simulink model "k1visbsp"  (Simulink 8.6)
settings: Solver=ode45  StartTime=0.0  StopTime=10.0  RelTol=1e-3
libraries: cdsEpicsOut x53, cdsTP x48, cdsFilt x30, cdsFiltCtrl x24, cdsEpicsStringIn x24, cdsRms x24, cdsIPCx x15, STATE_BIO_MASTER x3, cdsCDI64 x3, cdsCDO64 x3, VIS_LIB x2, cdsMuxMatrix x2
(part 1 of 4)
settings Model: Creator=controls  LastModifiedBy=controls
settings DataIOCC: SignalLoggingSaveFormat=Dataset
settings OptimizationCC: ExpressionDepthLimit=128
settings DebuggingCC: UnderspecifiedInitializationDetection=Simplified  MergeDetectMultiDrivingBlocksExec=error  SolverPrmCheckMsg=none  FcnCallInpInsideContextMsg=EnableAllAsError  StateNameClashWarn=none
settings GRTTargetCC: CombineOutputUpdateFcns=on  GRTInterface=off

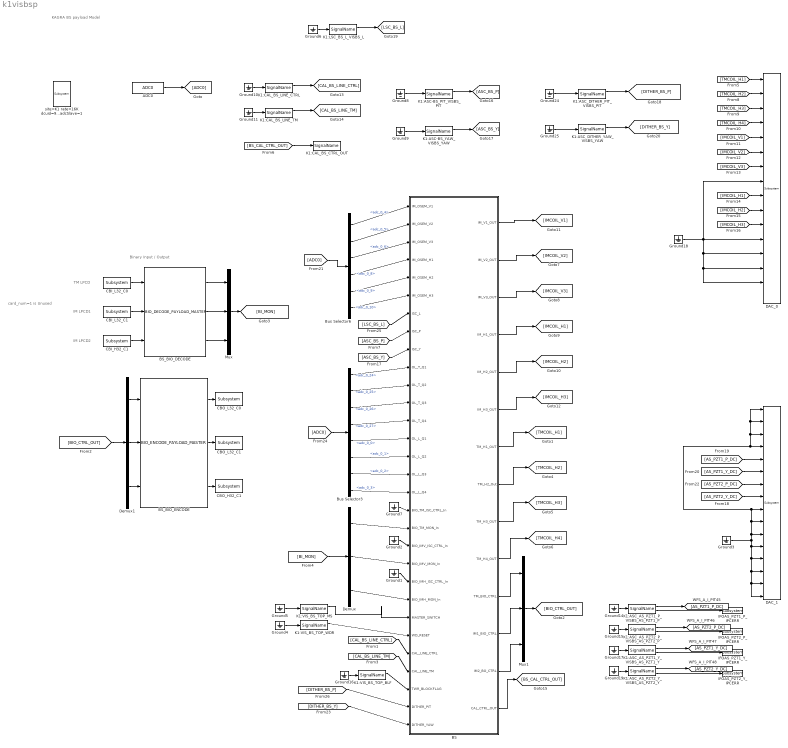
== system k1visbsp ==
  note: KAGRA BS payload Model
  note: TM LPCD
  note: Binary Input / Output
  note: card_num=1 is Unused
  note: IM LPCD1
  note: IM LPCD2
  ADC0 : cdsAdcx0/ADC0  Tag=cdsAdc  Description=|
      | type-GSC_16AI64SSA
      | card_num=0
      settings: AttributesFormatString=%<Description>\n%<Tag>
  BS : Subsystem  AncestorBlock=TYPEB_MASTER/TYPEB_PAYLOAD_shutdown
  BS_BIO_DECODE : TYPEB_MASTER/BIO_DECODE_PAYLOAD_MASTER
  BS_BIO_ENCODE : TYPEB_MASTER/BIO_ENCODE_PAYLOAD_MASTER
  Bus Selector3 : BusSelector  Description=ADC Selector  OutputSignals=adc_0_24,adc_0_25,adc_0_26,adc_0_27,adc_0_0,adc_0_1,adc_0_2,adc_0_3
      settings: AttributesFormatString=%<Description>
  Bus Selector6 : BusSelector  Description=ADC Selector  OutputSignals=adc_0_4,adc_0_5,adc_0_6,adc_0_8,adc_0_9,adc_0_10
      settings: AttributesFormatString=%<Description>
  CBI_H32_C1 : cdsCDI64/Subsystem  Tag=cdsCDI64  Description=card_num=3
      settings: AttributesFormatString=%<Tag>\n%<Description>
  CBI_L32_C0 : cdsCDI64/Subsystem  Tag=cdsCDI64  Description=card_num=0
      settings: AttributesFormatString=%<Tag>\n%<Description>
  CBI_L32_C1 : cdsCDI64/Subsystem  Tag=cdsCDI64  Description=card_num=2
      settings: AttributesFormatString=%<Tag>\n%<Description>
  CBO_H32_C1 : cdsCDO64/Subsystem  Tag=cdsCDO64  Description=card_num=3
      settings: AttributesFormatString=%<Tag>\n%<Description>
  CBO_L32_C0 : cdsCDO64/Subsystem  Tag=cdsCDO64  Description=card_num=0
      settings: AttributesFormatString=%<Tag>\n%<Description>
  CBO_L32_C1 : cdsCDO64/Subsystem  Tag=cdsCDO64  Description=card_num=2
      settings: AttributesFormatString=%<Tag>\n%<Description>
  DAC_0 : dac/Subsystem  Description=|
      | type=GSC_16AO16,
      | card_num=0
      settings: AttributesFormatString=%<Description>
  DAC_1 : dac/Subsystem  Description=|
      | type=GSC_16AO16,
      | card_num=1
      settings: AttributesFormatString=%<Description>
  Demux : Demux  Outputs=3
  Demux1 : Demux  Outputs=3
  Ground{1..11,14..19,24..25} (19 alike) : Ground
  IFOAS_PZT1_P_IPCERR : cdsEpicsOut/Subsystem  Tag=cdsEpicsOutput  Description=|
      | Purpose:                                          
      | Output a FE signal to an EPICS channel.           
      |                                                   
      | Operation:                                        
      | Takes input value and passes it to EPICS record.  
      |                                                   
      | Usage:                                            
      | Name the part with the desired EPICS rrecord name.
      settings: AttributesFormatString=%<Tag>
  IFOAS_PZT1_Y_IPCERR : cdsEpicsOut/Subsystem  Tag=cdsEpicsOutput  Description=|
      | Purpose:                                          
      | Output a FE signal to an EPICS channel.           
      |                                                   
      | Operation:                                        
      | Takes input value and passes it to EPICS record.  
      |                                                   
      | Usage:                                            
      | Name the part with the desired EPICS rrecord name.
      settings: AttributesFormatString=%<Tag>
  IFOAS_PZT2_P_IPCERR : cdsEpicsOut/Subsystem  Tag=cdsEpicsOutput  Description=|
      | Purpose:                                          
      | Output a FE signal to an EPICS channel.           
      |                                                   
      | Operation:                                        
      | Takes input value and passes it to EPICS record.  
      |                                                   
      | Usage:                                            
      | Name the part with the desired EPICS rrecord name.
      settings: AttributesFormatString=%<Tag>
  IFOAS_PZT2_Y_IPCERR : cdsEpicsOut/Subsystem  Tag=cdsEpicsOutput  Description=|
      | Purpose:                                          
      | Output a FE signal to an EPICS channel.           
      |                                                   
      | Operation:                                        
      | Takes input value and passes it to EPICS record.  
      |                                                   
      | Usage:                                            
      | Name the part with the desired EPICS rrecord name.
      settings: AttributesFormatString=%<Tag>
  K1:ASC-BS_PIT_VISBS_PIT : cdsIPCx/SignalName  Tag=cdsIPCx_PCIE  Description=Inter-Process Communication via PCI Express network.
      settings: AttributesFormatString=%<Tag>
  K1:ASC-BS_YAW_VISBS_YAW : cdsIPCx/SignalName  Tag=cdsIPCx_PCIE  Description=Inter-Process Communication via PCI Express network.
      settings: AttributesFormatString=%<Tag>
  K1:ASC_AS_PZT1_P_VISBS_AS_PZT1_P : cdsIPCx/SignalName  Tag=cdsIPCx_PCIE  Description=Inter-Process Communication via PCI Express network.
      settings: AttributesFormatString=%<Tag>
  K1:ASC_AS_PZT1_Y_VISBS_AS_PZT1_Y : cdsIPCx/SignalName  Tag=cdsIPCx_PCIE  Description=Inter-Process Communication via PCI Express network.
      settings: AttributesFormatString=%<Tag>
  K1:ASC_AS_PZT2_P_VISBS_AS_PZT2_P : cdsIPCx/SignalName  Tag=cdsIPCx_PCIE  Description=Inter-Process Communication via PCI Express network.
      settings: AttributesFormatString=%<Tag>
  K1:ASC_AS_PZT2_Y_VISBS_AS_PZT2_Y : cdsIPCx/SignalName  Tag=cdsIPCx_PCIE  Description=Inter-Process Communication via PCI Express network.
      settings: AttributesFormatString=%<Tag>
  K1:ASC_DITHER_PIT_VISBS_PIT : cdsIPCx/SignalName  Tag=cdsIPCx_PCIE  Description=Inter-Process Communication via PCI Express network.
      settings: AttributesFormatString=%<Tag>
  K1:ASC_DITHER_YAW_VISBS_YAW : cdsIPCx/SignalName  Tag=cdsIPCx_PCIE  Description=Inter-Process Communication via PCI Express network.
      settings: AttributesFormatString=%<Tag>
  K1:CAL_BS_CTRL_OUT : cdsIPCx/SignalName  Tag=cdsIPCx_PCIE  Description=Inter-Process Communication via PCI Express network.
      settings: AttributesFormatString=%<Tag>
  K1:CAL_BS_LINE_CTRL : cdsIPCx/SignalName  Tag=cdsIPCx_PCIE  Description=Inter-Process Communication via PCI Express network.
      settings: AttributesFormatString=%<Tag>
  K1:CAL_BS_LINE_TM : cdsIPCx/SignalName  Tag=cdsIPCx_PCIE  Description=Inter-Process Communication via PCI Express network.
      settings: AttributesFormatString=%<Tag>
  K1:LSC_BS_L_VISBS_L : cdsIPCx/SignalName  Tag=cdsIPCx_PCIE  Description=Inter-Process Communication via PCI Express network.
      settings: AttributesFormatString=%<Tag>
  K1:VIS_BS_TOP_BLF : cdsIPCx/SignalName  Tag=cdsIPCx_SHMEM  Description=Inter-Process Communication via Shared memory.
      settings: AttributesFormatString=%<Tag>
  K1:VIS_BS_TOP_MS : cdsIPCx/SignalName  Tag=cdsIPCx_SHMEM  Description=Inter-Process Communication via Shared memory.
      settings: AttributesFormatString=%<Tag>
  K1:VIS_BS_TOP_WDR : cdsIPCx/SignalName  Tag=cdsIPCx_SHMEM  Description=Inter-Process Communication via Shared memory.
      settings: AttributesFormatString=%<Tag>
  Mux : Mux  Inputs=3
  Mux1 : Mux  Inputs=3
  site=K1 rate=16K dcuid=92 host=k1bs specific_cpu=5 adcSlave=1 : cdsParameters/Subsystem  Tag=cdsParameters  Description=|
      | Purpose:                                                                                                                                                                                                                                
      | Provide system parameters to the FE code generator to properly configure the generated EPICS names, rep rate of the FE controller, and the Data Acquisition node ID for proper storage of data from this FE controller.                 
      |                                                                                                                                                                                                                                         
      | Useage:                                                                                                                                                                                                                                 
      | The part NAME field is used to identify the FE parameters. It must be of the form:                                                                                                                                                      
      | site=                                                                                                                                                                                                                                   
      | rate=                                                                                                                                                                                                                                   
      | dcuid=                                                                                                                                                                                                                                  
      |                                                                                                                                                                                                                                         
      | Where:                                                                                                                                                                                                                                  
      | site= argument may be H1, H2, L1, M1, G1, either as a single argument or multiple, for example site=H1,H2. These are the only names allowed. These will become the first two characters of all EPICS and signal names (for example G1:).
      |                                                                                                                                                                                                                                         
      | rate= may be 2K, 16K, 32K, or 64K                                                                                                                                                                                                       
      |                                                                                                                                                                                                                                         
      | dcuid= is site specific ie it must be unique at each site.
      settings: AttributesFormatString=%<Tag>
  wires:
  ADC0/1 -> [ADC0]
  [ADC0] -> Bus Selector6/1
  BS/10(TM_H4_OUT) -> [TMCOIL_H4]
  BS/9(TM_H3_OUT) -> [TMCOIL_H3]
  BS/8(TM_H2_Out) -> [TMCOIL_H2]
  BS/7(TM_H1_OUT) -> [TMCOIL_H1]
  BS/1(IM_V1_OUT) -> [IMCOIL_V1]
  BS/2(IM_V2_OUT) -> [IMCOIL_V2]
  BS/3(IM_V3_OUT) -> [IMCOIL_V3]
  BS/4(IM_H1_OUT) -> [IMCOIL_H1]
  BS/5(IM_H2_OUT) -> [IMCOIL_H2]
  BS/6(IM_H3_OUT) -> [IMCOIL_H3]
  Ground18/1 -> DAC_0/12, DAC_0/13, DAC_0/14, DAC_0/15, DAC_0/8
  Bus Selector6/1 -> BS/1(IM_OSEM_V1)  "<adc_0_4>"
  Bus Selector6/2 -> BS/2(IM_OSEM_V2)  "<adc_0_5>"
  Bus Selector6/3 -> BS/3(IM_OSEM_V3)  "<adc_0_6>"
  [TMCOIL_H2] -> DAC_0/2
  [TMCOIL_H3] -> DAC_0/3
  [TMCOIL_H1] -> DAC_0/1
  [TMCOIL_H4] -> DAC_0/4
  [IMCOIL_V1] -> DAC_0/5
  [IMCOIL_V2] -> DAC_0/6
  [IMCOIL_V3] -> DAC_0/7
  Bus Selector6/4 -> BS/4(IM_OSEM_H1)  "<adc_0_8>"
  Bus Selector6/5 -> BS/5(IM_OSEM_H2)  "<adc_0_9>"
  Bus Selector6/6 -> BS/6(IM_OSEM_H3)  "<adc_0_10>"
  [IMCOIL_H3] -> DAC_0/11
  [IMCOIL_H2] -> DAC_0/10
  [IMCOIL_H1] -> DAC_0/9
  [LSC_BS_L] -> BS/7(ISC_L)
  [ADC0] -> Bus Selector3/1
  Bus Selector3/1 -> BS/10(OL_T_Q1)  "<adc_0_24>"
  Bus Selector3/2 -> BS/11(OL_T_Q2)  "<adc_0_25>"
  Bus Selector3/3 -> BS/12(OL_T_Q3)  "<adc_0_26>"
  Bus Selector3/4 -> BS/13(OL_T_Q4)  "<adc_0_27>"
  BS_BIO_ENCODE/1 -> CBO_L32_C0/1
  BS_BIO_ENCODE/3 -> CBO_H32_C1/1
  BS_BIO_ENCODE/2 -> CBO_L32_C1/1
  CBI_L32_C0/1 -> BS_BIO_DECODE/1
  CBI_L32_C1/1 -> BS_BIO_DECODE/2
  CBI_H32_C1/1 -> BS_BIO_DECODE/3
  BS_BIO_DECODE/2 -> Mux/2
  BS_BIO_DECODE/3 -> Mux/3
  BS_BIO_DECODE/1 -> Mux/1
  Mux/1 -> [BI_MON]
  Demux1/2 -> BS_BIO_ENCODE/2
  Demux1/3 -> BS_BIO_ENCODE/3
  Demux1/1 -> BS_BIO_ENCODE/1
  [BIO_CTRL_OUT] -> Demux1/1
  Mux1/1 -> [BIO_CTRL_OUT]
  [BI_MON] -> Demux/1
  Demux/1 -> BS/19(BIO_TM_MON_In)
  Demux/2 -> BS/21(BIO_IMV_MON_In)
  Demux/3 -> BS/23(BIO_IMH_MON_In)
  Ground7/1 -> BS/18(BIO_TM_ISC_CTRL_In)
  Ground1/1 -> BS/22(BIO_IMH_ISC_CTRL_In)
  Ground2/1 -> BS/20(BIO_IMV_ISC_CTRL_In)
  Ground4/1 -> K1:VIS_BS_TOP_WDR/1
  Ground5/1 -> K1:VIS_BS_TOP_MS/1
  K1:VIS_BS_TOP_WDR/1 -> BS/25(WD_RESET)
  K1:VIS_BS_TOP_MS/1 -> BS/24(MASTER_SWITCH)
  Ground10/1 -> K1:CAL_BS_LINE_CTRL/1
  K1:CAL_BS_LINE_CTRL/1 -> [CAL_BS_LINE_CTRL]
  Ground11/1 -> K1:CAL_BS_LINE_TM/1
  K1:CAL_BS_LINE_TM/1 -> [CAL_BS_LINE_TM]
  [CAL_BS_LINE_CTRL] -> BS/26(CAL_LINE_CTRL)
  [CAL_BS_LINE_TM] -> BS/27(CAL_LINE_TM)
  BS/14(CAL_CTRL_OUT) -> [BS_CAL_CTRL_OUT]
  [BS_CAL_CTRL_OUT] -> K1:CAL_BS_CTRL_OUT/1
  Ground3/1 -> DAC_1/13, DAC_1/14, DAC_1/15, DAC_1/16, DAC_1/12, DAC_1/1, DAC_1/2, DAC_1/3, DAC_1/4, DAC_1/9, DAC_1/10, DAC_1/11
  Bus Selector3/5 -> BS/14(OL_L_Q1)  "<adc_0_0>"
  Bus Selector3/6 -> BS/15(OL_L_Q2)  "<adc_0_1>"
  Bus Selector3/7 -> BS/16(OL_L_Q3)  "<adc_0_2>"
  Bus Selector3/8 -> BS/17(OL_L_Q4)  "<adc_0_3>"
  [ASC_BS_P] -> BS/8(ISC_P)
  [ASC_BS_Y] -> BS/9(ISC_Y)
  Ground16/1 -> K1:VIS_BS_TOP_BLF/1
  K1:VIS_BS_TOP_BLF/1 -> BS/28(TWR_BLOCKFLAG)
  BS/11(TM_BIO_CTRL) -> Mux1/1
  BS/12(IM1_BIO_CTRL) -> Mux1/2
  BS/13(IM2_BO_CTRL) -> Mux1/3
  [DITHER_BS_Y] -> BS/30(DITHER_YAW)
  K1:ASC_AS_PZT1_P_VISBS_AS_PZT1_P/2 -> IFOAS_PZT1_P_IPCERR/1
  K1:ASC_AS_PZT2_P_VISBS_AS_PZT2_P/2 -> IFOAS_PZT2_P_IPCERR/1
  K1:ASC_AS_PZT1_Y_VISBS_AS_PZT1_Y/2 -> IFOAS_PZT1_Y_IPCERR/1
  K1:ASC_AS_PZT2_Y_VISBS_AS_PZT2_Y/2 -> IFOAS_PZT2_Y_IPCERR/1
  K1:ASC_AS_PZT1_P_VISBS_AS_PZT1_P/1 -> [AS_PZT1_P_DC]
  K1:ASC_AS_PZT2_P_VISBS_AS_PZT2_P/1 -> [AS_PZT2_P_DC]
  K1:ASC_AS_PZT1_Y_VISBS_AS_PZT1_Y/1 -> [AS_PZT1_Y_DC]
  K1:ASC_AS_PZT2_Y_VISBS_AS_PZT2_Y/1 -> [AS_PZT2_Y_DC]
  Ground14/1 -> K1:ASC_AS_PZT1_P_VISBS_AS_PZT1_P/1
  Ground15/1 -> K1:ASC_AS_PZT2_P_VISBS_AS_PZT2_P/1
  Ground17/1 -> K1:ASC_AS_PZT1_Y_VISBS_AS_PZT1_Y/1
  Ground19/1 -> K1:ASC_AS_PZT2_Y_VISBS_AS_PZT2_Y/1
  [AS_PZT2_Y_DC] -> DAC_1/8
  [AS_PZT2_P_DC] -> DAC_1/7
  [AS_PZT1_Y_DC] -> DAC_1/6
  [AS_PZT1_P_DC] -> DAC_1/5
  Ground6/1 -> K1:LSC_BS_L_VISBS_L/1
  K1:LSC_BS_L_VISBS_L/1 -> [LSC_BS_L]
  Ground8/1 -> K1:ASC-BS_PIT_VISBS_PIT/1
  Ground9/1 -> K1:ASC-BS_YAW_VISBS_YAW/1
  Ground25/1 -> K1:ASC_DITHER_YAW_VISBS_YAW/1
  Ground24/1 -> K1:ASC_DITHER_PIT_VISBS_PIT/1
  [DITHER_BS_P] -> BS/29(DITHER_PIT)
  K1:ASC-BS_PIT_VISBS_PIT/1 -> [ASC_BS_P]
  K1:ASC-BS_YAW_VISBS_YAW/1 -> [ASC_BS_Y]
  K1:ASC_DITHER_PIT_VISBS_PIT/1 -> [DITHER_BS_P]
  K1:ASC_DITHER_YAW_VISBS_YAW/1 -> [DITHER_BS_Y]

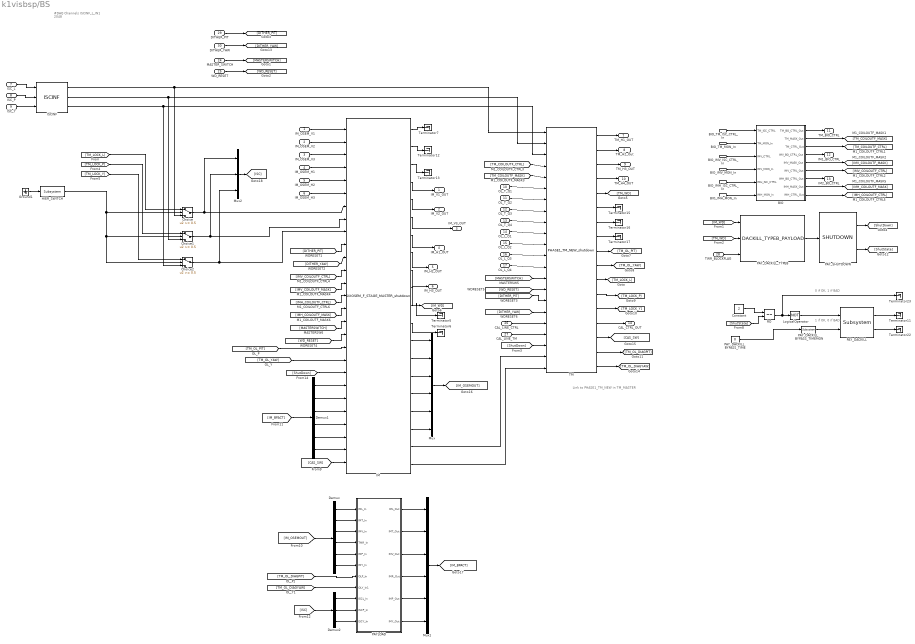
== system k1visbsp/BS ==
  note: #DAQ Channels
      | ISCINF_L_IN1 2048
  note: 1 if OK, 0 if BAD
  note: 0 if OK, 1 if BAD
  note: Link to PHASE1_TM_NEW in TM_MASTER
  IM_OSEM_V1 : Inport
  IM_OSEM_V2 : Inport  Port=2
  IM_OSEM_V3 : Inport  Port=3
  IM_OSEM_H1 : Inport  Port=4
  IM_OSEM_H2 : Inport  Port=5
  IM_OSEM_H3 : Inport  Port=6
  ISC_L : Inport  Port=7
  ISC_P : Inport  Port=8
  ISC_Y : Inport  Port=9
  OL_T_Q1 : Inport  Port=10
  OL_T_Q2 : Inport  Port=11
  OL_T_Q3 : Inport  Port=12
  OL_T_Q4 : Inport  Port=13
  OL_L_Q1 : Inport  Port=14
  OL_L_Q2 : Inport  Port=15
  OL_L_Q3 : Inport  Port=16
  OL_L_Q4 : Inport  Port=17
  BIO_TM_ISC_CTRL_In : Inport  Port=18
  BIO_TM_MON_In : Inport  Port=19
  BIO_IMV_ISC_CTRL_In : Inport  Port=20
  BIO_IMV_MON_In : Inport  Port=21
  BIO_IMH_ISC_CTRL_In : Inport  Port=22
  BIO_IMH_MON_In : Inport  Port=23
  MASTER_SWITCH : Inport  Port=24
  WD_RESET : Inport  Port=25
  CAL_LINE_CTRL : Inport  Port=26
  CAL_LINE_TM : Inport  Port=27
  TWR_BLOCKFLAG : Inport  Port=28
  DITHER_PIT : Inport  Port=29
  DITHER_YAW : Inport  Port=30
  BIO : Subsystem
  Choice : Switch  Threshold=0.5
  Choice1 : Switch  Threshold=0.5
  Choice2 : Switch  Threshold=0.5
  Constant : Constant  Value=2
  Demux : Demux  Outputs=6
  Demux1 : Demux  Outputs=6
  Demux2 : Demux  Outputs=3
  Ground1 : Ground
  HIER_SWITCH : cdsEpicsBinIn/Subsystem  Tag=cdsEpicsBinIn  Description=|
      | Purpose:                                                                            
      | Create an EPICS binary (0 or 1) input channel to the FE realtime controls.          
      |                                                                                     
      | Operation:                                                                          
      | Outputs value from an EPICS ai record. Value is binary input (bi Epics record type).
      |                                                                                     
      | Usage:                                                                              
      | Name the part with the desired EPICS channel name.
      settings: AttributesFormatString=%<Tag>
  IM : SIXOSEM_F_STAGE_MASTER/SIXOSEM_F_STAGE_MASTER_shutdown  Description=SIXOSEMSTAGE_FACE_MASTER
  ISCINF : VIS_LIB/ISCINF
  LogicalOperator : Logic  Operator=NOT  AllPortsSameDT=off  OutDataTypeStr=boolean
  Mux : Mux  Inputs=6
  Mux1 : Mux  Inputs=6
  Mux2 : Mux  Inputs=3
  PAYLOAD : Subsystem
  PAY_DACKILL : cdsDacKill/Subsystem  Description=cdsDacKill
      settings: AttributesFormatString=%<Description>
  PAY_DACKILL_BYPASS_TIME : Constant  Value=0
  PAY_DACKILL_BYPASS_TIMEMON : cdsEpicsOut/Subsystem  Tag=cdsEpicsOutput  Description=|
      | Purpose:                                          
      | Output a FE signal to an EPICS channel.           
      |                                                   
      | Operation:                                        
      | Takes input value and passes it to EPICS record.  
      |                                                   
      | Usage:                                            
      | Name the part with the desired EPICS rrecord name.
      settings: AttributesFormatString=%<Tag>
  PAY_DACKILL_TYPEB : VIS_LIB/DACKILL_TYPEB_PAYLOAD
  PAY_SHUTDOWN : SHUTDOWN/SHUTDOWN
  RO : RelationalOperator  Operator===  OutDataTypeStr=boolean
  TM : TM_MASTER/PHASE1_TM_NEW_shutdown
  Terminator{5..7,11..13,15..17,22..23} (11 alike) : Terminator
  IM_V1_OUT : Outport
  IM_V2_OUT : Outport  Port=2
  IM_V3_OUT : Outport  Port=3
  IM_H1_OUT : Outport  Port=4
  IM_H2_OUT : Outport  Port=5
  IM_H3_OUT : Outport  Port=6
  TM_H1_OUT : Outport  Port=7
  TM_H2_Out : Outport  Port=8
  TM_H3_OUT : Outport  Port=9
  TM_H4_OUT : Outport  Port=10
  TM_BIO_CTRL : Outport  Port=11
  IM1_BIO_CTRL : Outport  Port=12
  IM2_BO_CTRL : Outport  Port=13
  CAL_CTRL_OUT : Outport  Port=14
  wires:
  [ISC] -> Demux2/1
  Demux2/3 -> PAYLOAD/11(ISCY_In)
  Demux2/2 -> PAYLOAD/10(ISCP_In)
  Demux2/1 -> PAYLOAD/9(ISCL_In)
  Mux2/1 -> [ISC]
  [IM_BPACT] -> Demux1/1
  Demux1/1 -> IM/21
  Demux1/2 -> IM/22
  Demux1/3 -> IM/23
  Demux1/6 -> IM/26
  Demux1/4 -> IM/24
  Demux1/5 -> IM/25
  Mux1/1 -> [IM_BPACT]
  PAYLOAD/6(IMY_Out) -> Mux1/6
  PAYLOAD/5(IMP_Out) -> Mux1/5
  PAYLOAD/4(IMR_Out) -> Mux1/4
  PAYLOAD/3(IMV_Out) -> Mux1/3
  PAYLOAD/2(IMT_Out) -> Mux1/2
  PAYLOAD/1(IML_Out) -> Mux1/1
  [TM_OL_DIAGPIT] -> PAYLOAD/7(OLP_In)
  [TM_OL_DIAGYAW] -> PAYLOAD/8(OLY_In1)
  [IM_OSEMOUT] -> Demux/1
  Demux/1 -> PAYLOAD/1(IML_In)
  Demux/2 -> PAYLOAD/2(IMT_In)
  Demux/3 -> PAYLOAD/3(IMV_In)
  Demux/4 -> PAYLOAD/4(TMR_In)
  Demux/5 -> PAYLOAD/5(IMP_In)
  Demux/6 -> PAYLOAD/6(IMY_In)
  Mux/1 -> [IM_OSEMOUT]
  IM/18 -> Mux/6
  IM/17 -> Mux/5
  IM/16 -> Mux/4
  IM/15 -> Mux/3
  IM/14 -> Mux/2
  IM/13 -> Mux/1
  [CAS_SW] -> IM/27
  TM/15 -> [CAS_SW]
  [TM_LOCK_Y] -> Choice2/1
  [TM_LOCK_P] -> Choice1/1
  [TM_LOCK_L] -> Choice/1
  TM/11 -> [TM_LOCK_L]
  TM/12 -> [TM_LOCK_P]
  TM/13 -> [TM_LOCK_Y]
  HIER_SWITCH/1 -> Choice2/2, Choice1/2, Choice/2
  Ground1/1 -> HIER_SWITCH/1
  ISCINF/3 -> TM/3, Choice2/3
  ISCINF/2 -> TM/2, Choice1/3
  ISCINF/1 -> TM/1, Choice/3
  ISC_Y/1 -> ISCINF/3
  ISC_P/1 -> ISCINF/2
  ISC_L/1 -> ISCINF/1
  DITHER_YAW/1 -> [DITHER_YAW]
  DITHER_PIT/1 -> [DITHER_PIT]
  [DITHER_YAW] -> IM/11
  [DITHER_PIT] -> IM/10
  [DITHER_YAW] -> TM/17
  [DITHER_PIT] -> TM/16
  [IMV_COILOUTF_CTRL] -> IM/12
  [IMH_COILOUTF_CTRL] -> IM/14
  [IMV_COILOUTF_MASK] -> IM/13
  [IMH_COILOUTF_MASK] -> IM/15
  [MASTERSWITCH] -> IM/16
  [WD_RESET] -> IM/17
  [TM_OL_PIT] -> IM/18
  [TM_OL_YAW] -> IM/19
  [ShutDown] -> IM/20
  Choice2/1 -> IM/9, Mux2/3
  Choice1/1 -> IM/8, Mux2/2
  Choice/1 -> IM/7, Mux2/1
  IM_OSEM_H3/1 -> IM/6
  IM_OSEM_H2/1 -> IM/5
  IM_OSEM_H1/1 -> IM/4
  IM_OSEM_V3/1 -> IM/3
  IM_OSEM_V2/1 -> IM/2
  IM_OSEM_V1/1 -> IM/1
  PAY_SHUTDOWN/1 -> [ShutDown]
  RO/1 -> LogicalOperator/1, Terminator23/1
  [ShutState] -> RO/2
  Constant/1 -> RO/1
  PAY_SHUTDOWN/2 -> [ShutState]
  PAY_DACKILL_TYPEB/1 -> PAY_SHUTDOWN/1
  PAY_DACKILL/2 -> Terminator22/1
  PAY_DACKILL_BYPASS_TIMEMON/1 -> PAY_DACKILL/2
  PAY_DACKILL/1 -> Terminator11/1
  PAY_DACKILL_BYPASS_TIME/1 -> PAY_DACKILL_BYPASS_TIMEMON/1
  LogicalOperator/1 -> PAY_DACKILL/1
  [ShutDown] -> TM/20
  TM/14 -> CAL_CTRL_OUT/1
  TWR_BLOCKFLAG/1 -> PAY_DACKILL_TYPEB/3
  IM/1 -> Terminator7/1
  IM/12 -> Terminator6/1
  IM/5 -> IM_V2_OUT/1
  IM/6 -> IM_V3_OUT/1
  IM/7 -> IM_H1_OUT/1
  IM/8 -> IM_H2_OUT/1
  IM/9 -> IM_H3_OUT/1
  TM/1 -> TM_H1_OUT/1
  TM/3 -> TM_H3_OUT/1
  TM/2 -> TM_H2_Out/1
  TM/4 -> TM_H4_OUT/1
  IM/2 -> Terminator12/1
  TM/7 -> Terminator16/1
  TM/6 -> Terminator15/1
  TM/8 -> Terminator17/1
  OL_T_Q4/1 -> TM/9
  OL_T_Q1/1 -> TM/6
  OL_T_Q3/1 -> TM/8
  [MASTERSWITCH] -> TM/14
  OL_T_Q2/1 -> TM/7
  [TM_COILOUTF_CTRL] -> TM/4
  [WD_RESET] -> TM/15
  [TM_COILOUTF_MASK] -> TM/5
  IM/4 -> IM_V1_OUT/1
  IM/3 -> Terminator13/1
  TM/5 -> [TM_WD]
  IM/10 -> [IM_WD]
  OL_L_Q3/1 -> TM/12
  OL_L_Q4/1 -> TM/13
  OL_L_Q2/1 -> TM/11
  OL_L_Q1/1 -> TM/10
  TM/10 -> [TM_OL_YAW]
  TM/9 -> [TM_OL_PIT]
  IM/11 -> Terminator5/1
  [IM_WD] -> PAY_DACKILL_TYPEB/1
  [TM_WD] -> PAY_DACKILL_TYPEB/2
  BIO/8(IMH_MASK_Out) -> [IMH_COILOUTF_MASK]
  BIO_TM_MON_In/1 -> BIO/2(TM_MON_In)
  BIO/4(IMV_BO_CTRL_Out) -> IM1_BIO_CTRL/1
  BIO_TM_ISC_CTRL_In/1 -> BIO/1(TM_ISC_CTRL)
  BIO_IMV_ISC_CTRL_In/1 -> BIO/3(IMV_CTRL)
  BIO_IMV_MON_In/1 -> BIO/4(IMV_MON_In)
  BIO/1(TM_BO_CTRL_Out) -> TM_BIO_CTRL/1
  BIO/7(IMH_BO_CTRL_Out) -> IM2_BO_CTRL/1
  BIO/5(IMV_MASK_Out) -> [IMV_COILOUTF_MASK]
  BIO/6(IMV_CTRL_Out) -> [IMV_COILOUTF_CTRL]
  BIO/2(TM_MASK_Out) -> [TM_COILOUTF_MASK]
  BIO/3(TM_CTRL_Out) -> [TM_COILOUTF_CTRL]
  BIO/9(IMH_CTRL_Out) -> [IMH_COILOUTF_CTRL]
  BIO_IMH_ISC_CTRL_In/1 -> BIO/5(IMH_ISC_CTRL)
  BIO_IMH_MON_In/1 -> BIO/6(IMH_MON_In)
  MASTER_SWITCH/1 -> [MASTERSWITCH]
  WD_RESET/1 -> [WD_RESET]
  CAL_LINE_CTRL/1 -> TM/18
  CAL_LINE_TM/1 -> TM/19
  IM/19 -> TM/21
  IM/20 -> TM/22
  TM/16 -> [TM_OL_DIAGPIT]
  TM/17 -> [TM_OL_DIAGYAW]

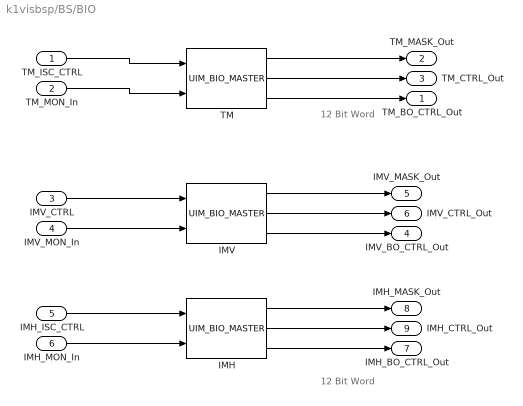
== system k1visbsp/BS/BIO ==
  note: 12 Bit Word
  note: 12 Bit Word
  TM_ISC_CTRL : Inport
  TM_MON_In : Inport  Port=2
  IMV_CTRL : Inport  Port=3
  IMV_MON_In : Inport  Port=4
  IMH_ISC_CTRL : Inport  Port=5
  IMH_MON_In : Inport  Port=6
  IMH : STATE_BIO_MASTER/UIM_BIO_MASTER
  IMV : STATE_BIO_MASTER/UIM_BIO_MASTER
  TM : STATE_BIO_MASTER/UIM_BIO_MASTER
  TM_BO_CTRL_Out : Outport
  TM_MASK_Out : Outport  Port=2
  TM_CTRL_Out : Outport  Port=3
  IMV_BO_CTRL_Out : Outport  Port=4
  IMV_MASK_Out : Outport  Port=5
  IMV_CTRL_Out : Outport  Port=6
  IMH_BO_CTRL_Out : Outport  Port=7
  IMH_MASK_Out : Outport  Port=8
  IMH_CTRL_Out : Outport  Port=9
  wires:
  IMH/3 -> IMH_BO_CTRL_Out/1
  IMH/2 -> IMH_CTRL_Out/1
  IMH/1 -> IMH_MASK_Out/1
  IMV/3 -> IMV_BO_CTRL_Out/1
  IMV/1 -> IMV_MASK_Out/1
  IMV/2 -> IMV_CTRL_Out/1
  TM/2 -> TM_CTRL_Out/1
  TM/3 -> TM_BO_CTRL_Out/1
  TM/1 -> TM_MASK_Out/1
  IMH_ISC_CTRL/1 -> IMH/1
  IMV_MON_In/1 -> IMV/2
  IMH_MON_In/1 -> IMH/2
  TM_ISC_CTRL/1 -> TM/1
  IMV_CTRL/1 -> IMV/1
  TM_MON_In/1 -> TM/2

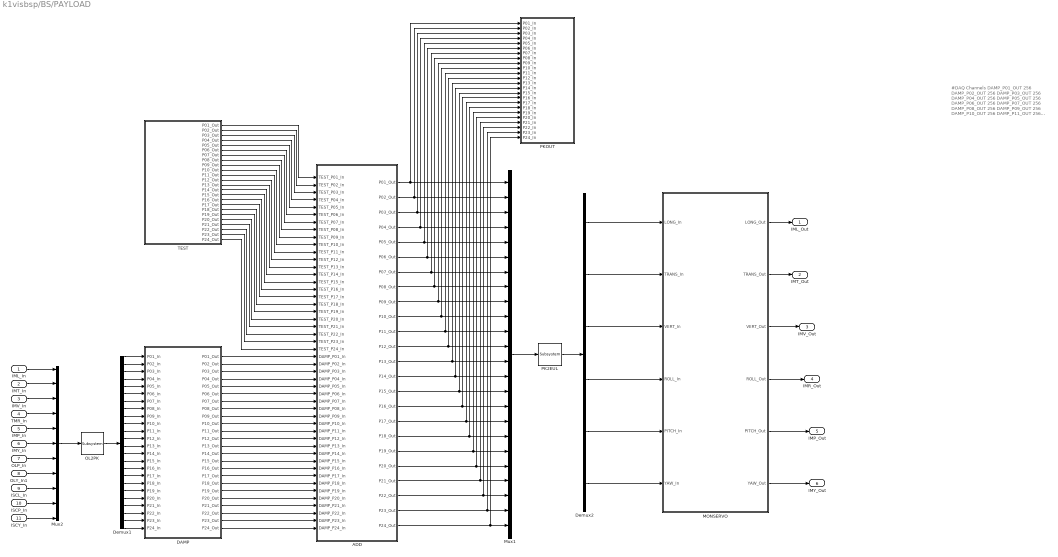
== system k1visbsp/BS/PAYLOAD ==
  note: #DAQ Channels
      | DAMP_P01_OUT 256
      | DAMP_P02_OUT 256
      | DAMP_P03_OUT 256
      | DAMP_P04_OUT 256
      | DAMP_P05_OUT 256
      | DAMP_P06_OUT 256
      | DAMP_P07_OUT 256
      | DAMP_P08_OUT 256
      | DAMP_P09_OUT 256
      | DAMP_P10_OUT 256
      | DAMP_P11_OUT 256
      | DAMP_P12_OUT 256
      | DAMP_P13_OUT 256
      | DAMP_P14_OUT 256
      | DAMP_P15_OUT 256
      | DAMP_P16_OUT 256
      | DAMP_P17_OUT 256
      | DAMP_P18_OUT 256
      | DAMP_P19_OUT 256
      | DAMP_P20_OUT 256
      | DAMP_P21_OUT 256
      | DAMP_P22_OUT 256
      | DAMP_P23_OUT 256
      | DAMP_P24_OUT 256
  IML_In : Inport
  IMT_In : Inport  Port=2
  IMV_In : Inport  Port=3
  TMR_In : Inport  Port=4
  IMP_In : Inport  Port=5
  IMY_In : Inport  Port=6
  OLP_In : Inport  Port=7
  OLY_In1 : Inport  Port=8
  ISCL_In : Inport  Port=9
  ISCP_In : Inport  Port=10
  ISCY_In : Inport  Port=11
  ADD : Subsystem
  DAMP : Subsystem
  Demux1 : Demux  Outputs=24
  Demux2 : Demux  Outputs=6
  MONSERVO : Subsystem
  Mux1 : Mux  Inputs=24
  Mux2 : Mux  Inputs=11
  OL2PK : cdsMuxMatrix/Subsystem  Tag=cdsMuxMatrix  Description=Any size matrix. Inputs and outputs must be connected using Mux and Demux parts.
      settings: AttributesFormatString=%<Tag>
  PK2EUL : cdsMuxMatrix/Subsystem  Tag=cdsMuxMatrix  Description=Any size matrix. Inputs and outputs must be connected using Mux and Demux parts.
      settings: AttributesFormatString=%<Tag>
  PKOUT : Subsystem
  TEST : Subsystem
  IML_Out : Outport
  IMT_Out : Outport  Port=2
  IMV_Out : Outport  Port=3
  IMR_Out : Outport  Port=4
  IMP_Out : Outport  Port=5
  IMY_Out : Outport  Port=6
  wires:
  MONSERVO/6(YAW_Out) -> IMY_Out/1
  MONSERVO/5(PITCH_Out) -> IMP_Out/1
  MONSERVO/4(ROLL_Out) -> IMR_Out/1
  MONSERVO/3(VERT_Out) -> IMV_Out/1
  MONSERVO/2(TRANS_Out) -> IMT_Out/1
  MONSERVO/1(LONG_Out) -> IML_Out/1
  ISCL_In/1 -> Mux2/9
  ISCP_In/1 -> Mux2/10
  ISCY_In/1 -> Mux2/11
  OLP_In/1 -> Mux2/7
  IMY_In/1 -> Mux2/6
  TMR_In/1 -> Mux2/4
  IMP_In/1 -> Mux2/5
  IML_In/1 -> Mux2/1
  IMT_In/1 -> Mux2/2
  IMV_In/1 -> Mux2/3
  Mux2/1 -> OL2PK/1
  OL2PK/1 -> Demux1/1
  Demux1/3 -> DAMP/3(P03_In)
  Demux1/6 -> DAMP/6(P06_In)
  Demux1/4 -> DAMP/4(P04_In)
  Demux1/1 -> DAMP/1(P01_In)
  Demux1/2 -> DAMP/2(P02_In)
  Demux1/7 -> DAMP/7(P07_In)
  Demux1/8 -> DAMP/8(P08_In)
  Demux1/9 -> DAMP/9(P09_In)
  Demux1/10 -> DAMP/10(P10_In)
  Demux1/11 -> DAMP/11(P11_In)
  Demux1/12 -> DAMP/12(P12_In)
  Demux1/5 -> DAMP/5(P05_In)
  TEST/12(P12_Out) -> ADD/12(TEST_P12_In)
  TEST/6(P06_Out) -> ADD/6(TEST_P06_In)
  TEST/7(P07_Out) -> ADD/7(TEST_P07_In)
  TEST/8(P08_Out) -> ADD/8(TEST_P08_In)
  TEST/9(P09_Out) -> ADD/9(TEST_P09_In)
  TEST/10(P10_Out) -> ADD/10(TEST_P10_In)
  TEST/11(P11_Out) -> ADD/11(TEST_P11_In)
  TEST/1(P01_Out) -> ADD/1(TEST_P01_In)
  TEST/2(P02_Out) -> ADD/2(TEST_P02_In)
  TEST/3(P03_Out) -> ADD/3(TEST_P03_In)
  TEST/4(P04_Out) -> ADD/4(TEST_P04_In)
  TEST/5(P05_Out) -> ADD/5(TEST_P05_In)
  DAMP/11(P11_Out) -> ADD/35(DAMP_P11_In)
  DAMP/4(P04_Out) -> ADD/28(DAMP_P04_In)
  DAMP/5(P05_Out) -> ADD/29(DAMP_P05_In)
  DAMP/6(P06_Out) -> ADD/30(DAMP_P06_In)
  DAMP/12(P12_Out) -> ADD/36(DAMP_P12_In)
  DAMP/8(P08_Out) -> ADD/32(DAMP_P08_In)
  DAMP/10(P10_Out) -> ADD/34(DAMP_P10_In)
  DAMP/7(P07_Out) -> ADD/31(DAMP_P07_In)
  DAMP/9(P09_Out) -> ADD/33(DAMP_P09_In)
  DAMP/1(P01_Out) -> ADD/25(DAMP_P01_In)
  DAMP/2(P02_Out) -> ADD/26(DAMP_P02_In)
  DAMP/3(P03_Out) -> ADD/27(DAMP_P03_In)
  Mux1/1 -> PK2EUL/1
  PK2EUL/1 -> Demux2/1
  Demux1/13 -> DAMP/13(P13_In)
  Demux1/14 -> DAMP/14(P14_In)
  Demux1/15 -> DAMP/15(P15_In)
  Demux1/16 -> DAMP/16(P16_In)
  Demux1/17 -> DAMP/17(P17_In)
  Demux1/18 -> DAMP/18(P18_In)
  Demux1/19 -> DAMP/19(P19_In)
  Demux1/20 -> DAMP/20(P20_In)
  Demux1/21 -> DAMP/21(P21_In)
  Demux1/22 -> DAMP/22(P22_In)
  Demux1/23 -> DAMP/23(P23_In)
  Demux1/24 -> DAMP/24(P24_In)
  TEST/13(P13_Out) -> ADD/13(TEST_P13_In)
  TEST/14(P14_Out) -> ADD/14(TEST_P14_In)
  TEST/15(P15_Out) -> ADD/15(TEST_P15_In)
  TEST/16(P16_Out) -> ADD/16(TEST_P16_In)
  TEST/17(P17_Out) -> ADD/17(TEST_P17_In)
  TEST/18(P18_Out) -> ADD/18(TEST_P18_In)
  TEST/19(P19_Out) -> ADD/19(TEST_P19_In)
  TEST/20(P20_Out) -> ADD/20(TEST_P20_In)
  TEST/21(P21_Out) -> ADD/21(TEST_P21_In)
  TEST/22(P22_Out) -> ADD/22(TEST_P22_In)
  TEST/23(P23_Out) -> ADD/23(TEST_P23_In)
  TEST/24(P24_Out) -> ADD/24(TEST_P24_In)
  DAMP/13(P13_Out) -> ADD/37(DAMP_P13_In)
  DAMP/14(P14_Out) -> ADD/38(DAMP_P14_In)
  DAMP/15(P15_Out) -> ADD/39(DAMP_P15_In)
  DAMP/16(P16_Out) -> ADD/40(DAMP_P16_In)
  DAMP/17(P17_Out) -> ADD/41(DAMP_P17_In)
  DAMP/18(P18_Out) -> ADD/42(DAMP_P18_In)
  DAMP/19(P19_Out) -> ADD/43(DAMP_P19_In)
  DAMP/20(P20_Out) -> ADD/44(DAMP_P20_In)
  DAMP/21(P21_Out) -> ADD/45(DAMP_P21_In)
  DAMP/22(P22_Out) -> ADD/46(DAMP_P22_In)
  DAMP/23(P23_Out) -> ADD/47(DAMP_P23_In)
  DAMP/24(P24_Out) -> ADD/48(DAMP_P24_In)
  ADD/16(P16_Out) -> PKOUT/16(P16_In), Mux1/16
  ADD/14(P14_Out) -> PKOUT/14(P14_In), Mux1/14
  ADD/19(P19_Out) -> PKOUT/19(P19_In), Mux1/19
  ADD/20(P20_Out) -> PKOUT/20(P20_In), Mux1/20
  ADD/24(P24_Out) -> PKOUT/24(P24_In), Mux1/24
  ADD/22(P22_Out) -> PKOUT/22(P22_In), Mux1/22
  ADD/23(P23_Out) -> PKOUT/23(P23_In), Mux1/23
  ADD/13(P13_Out) -> PKOUT/13(P13_In), Mux1/13
  ADD/15(P15_Out) -> PKOUT/15(P15_In), Mux1/15
  ADD/2(P02_Out) -> PKOUT/2(P02_In), Mux1/2
  ADD/3(P03_Out) -> PKOUT/3(P03_In), Mux1/3
  ADD/4(P04_Out) -> PKOUT/4(P04_In), Mux1/4
  ADD/5(P05_Out) -> PKOUT/5(P05_In), Mux1/5
  ADD/6(P06_Out) -> PKOUT/6(P06_In), Mux1/6
  ADD/7(P07_Out) -> PKOUT/7(P07_In), Mux1/7
  ADD/8(P08_Out) -> PKOUT/8(P08_In), Mux1/8
  ADD/9(P09_Out) -> PKOUT/9(P09_In), Mux1/9
  ADD/10(P10_Out) -> PKOUT/10(P10_In), Mux1/10
  ADD/11(P11_Out) -> PKOUT/11(P11_In), Mux1/11
  ADD/12(P12_Out) -> PKOUT/12(P12_In), Mux1/12
  ADD/17(P17_Out) -> PKOUT/17(P17_In), Mux1/17
  ADD/18(P18_Out) -> PKOUT/18(P18_In), Mux1/18
  ADD/21(P21_Out) -> PKOUT/21(P21_In), Mux1/21
  ADD/1(P01_Out) -> PKOUT/1(P01_In), Mux1/1
  Demux2/1 -> MONSERVO/1(LONG_In)
  Demux2/2 -> MONSERVO/2(TRANS_In)
  Demux2/3 -> MONSERVO/3(VERT_In)
  Demux2/4 -> MONSERVO/4(ROLL_In)
  Demux2/5 -> MONSERVO/5(PITCH_In)
  Demux2/6 -> MONSERVO/6(YAW_In)
  OLY_In1/1 -> Mux2/8

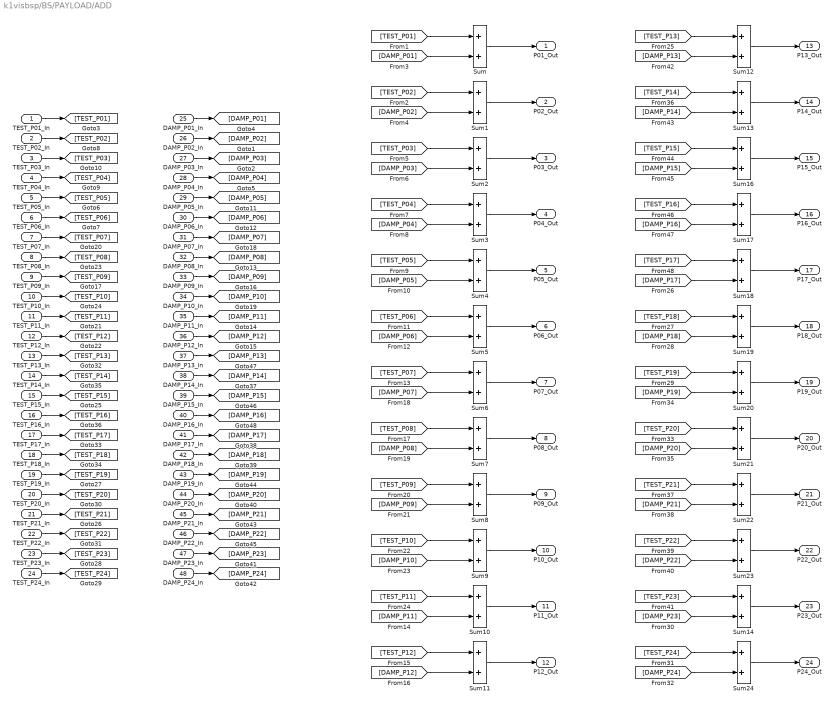
== system k1visbsp/BS/PAYLOAD/ADD ==
  TEST_P01_In : Inport
  TEST_P02_In : Inport  Port=2
  TEST_P03_In : Inport  Port=3
  TEST_P04_In : Inport  Port=4
  TEST_P05_In : Inport  Port=5
  TEST_P06_In : Inport  Port=6
  TEST_P07_In : Inport  Port=7
  TEST_P08_In : Inport  Port=8
  TEST_P09_In : Inport  Port=9
  TEST_P10_In : Inport  Port=10
  TEST_P11_In : Inport  Port=11
  TEST_P12_In : Inport  Port=12
  TEST_P13_In : Inport  Port=13
  TEST_P14_In : Inport  Port=14
  TEST_P15_In : Inport  Port=15
  TEST_P16_In : Inport  Port=16
  TEST_P17_In : Inport  Port=17
  TEST_P18_In : Inport  Port=18
  TEST_P19_In : Inport  Port=19
  TEST_P20_In : Inport  Port=20
  TEST_P21_In : Inport  Port=21
  TEST_P22_In : Inport  Port=22
  TEST_P23_In : Inport  Port=23
  TEST_P24_In : Inport  Port=24
  DAMP_P01_In : Inport  Port=25
  DAMP_P02_In : Inport  Port=26
  DAMP_P03_In : Inport  Port=27
  DAMP_P04_In : Inport  Port=28
  DAMP_P05_In : Inport  Port=29
  DAMP_P06_In : Inport  Port=30
  DAMP_P07_In : Inport  Port=31
  DAMP_P08_In : Inport  Port=32
  DAMP_P09_In : Inport  Port=33
  DAMP_P10_In : Inport  Port=34
  DAMP_P11_In : Inport  Port=35
  DAMP_P12_In : Inport  Port=36
  DAMP_P13_In : Inport  Port=37
  DAMP_P14_In : Inport  Port=38
  DAMP_P15_In : Inport  Port=39
  DAMP_P16_In : Inport  Port=40
  DAMP_P17_In : Inport  Port=41
  DAMP_P18_In : Inport  Port=42
  DAMP_P19_In : Inport  Port=43
  DAMP_P20_In : Inport  Port=44
  DAMP_P21_In : Inport  Port=45
  DAMP_P22_In : Inport  Port=46
  DAMP_P23_In : Inport  Port=47
  DAMP_P24_In : Inport  Port=48
  Sum{,1..14,16..24} (24 alike) : Sum
  P01_Out : Outport
  P02_Out : Outport  Port=2
  P03_Out : Outport  Port=3
  P04_Out : Outport  Port=4
  P05_Out : Outport  Port=5
  P06_Out : Outport  Port=6
  P07_Out : Outport  Port=7
  P08_Out : Outport  Port=8
  P09_Out : Outport  Port=9
  P10_Out : Outport  Port=10
  P11_Out : Outport  Port=11
  P12_Out : Outport  Port=12
  P13_Out : Outport  Port=13
  P14_Out : Outport  Port=14
  P15_Out : Outport  Port=15
  P16_Out : Outport  Port=16
  P17_Out : Outport  Port=17
  P18_Out : Outport  Port=18
  P19_Out : Outport  Port=19
  P20_Out : Outport  Port=20
  P21_Out : Outport  Port=21
  P22_Out : Outport  Port=22
  P23_Out : Outport  Port=23
  P24_Out : Outport  Port=24
  wires:
  DAMP_P02_In/1 -> [DAMP_P02]
  DAMP_P01_In/1 -> [DAMP_P01]
  [DAMP_P01] -> Sum/2
  [TEST_P01] -> Sum/1
  Sum/1 -> P01_Out/1
  DAMP_P03_In/1 -> [DAMP_P03]
  TEST_P01_In/1 -> [TEST_P01]
  TEST_P02_In/1 -> [TEST_P02]
  TEST_P03_In/1 -> [TEST_P03]
  TEST_P04_In/1 -> [TEST_P04]
  TEST_P05_In/1 -> [TEST_P05]
  TEST_P06_In/1 -> [TEST_P06]
  DAMP_P05_In/1 -> [DAMP_P05]
  DAMP_P04_In/1 -> [DAMP_P04]
  DAMP_P06_In/1 -> [DAMP_P06]
  DAMP_P08_In/1 -> [DAMP_P08]
  DAMP_P07_In/1 -> [DAMP_P07]
  DAMP_P09_In/1 -> [DAMP_P09]
  DAMP_P11_In/1 -> [DAMP_P11]
  DAMP_P10_In/1 -> [DAMP_P10]
  DAMP_P12_In/1 -> [DAMP_P12]
  TEST_P07_In/1 -> [TEST_P07]
  TEST_P08_In/1 -> [TEST_P08]
  TEST_P09_In/1 -> [TEST_P09]
  TEST_P10_In/1 -> [TEST_P10]
  TEST_P11_In/1 -> [TEST_P11]
  TEST_P12_In/1 -> [TEST_P12]
  [DAMP_P02] -> Sum1/2
  [TEST_P02] -> Sum1/1
  Sum1/1 -> P02_Out/1
  [DAMP_P03] -> Sum2/2
  [TEST_P03] -> Sum2/1
  Sum2/1 -> P03_Out/1
  [DAMP_P04] -> Sum3/2
  [TEST_P04] -> Sum3/1
  Sum3/1 -> P04_Out/1
  [DAMP_P05] -> Sum4/2
  [TEST_P05] -> Sum4/1
  Sum4/1 -> P05_Out/1
  [DAMP_P06] -> Sum5/2
  [TEST_P06] -> Sum5/1
  Sum5/1 -> P06_Out/1
  [DAMP_P07] -> Sum6/2
  [TEST_P07] -> Sum6/1
  Sum6/1 -> P07_Out/1
  [DAMP_P08] -> Sum7/2
  [TEST_P08] -> Sum7/1
  Sum7/1 -> P08_Out/1
  [DAMP_P09] -> Sum8/2
  [TEST_P09] -> Sum8/1
  Sum8/1 -> P09_Out/1
  [DAMP_P10] -> Sum9/2
  [TEST_P10] -> Sum9/1
  Sum9/1 -> P10_Out/1
  [DAMP_P11] -> Sum10/2
  [TEST_P11] -> Sum10/1
  Sum10/1 -> P11_Out/1
  [DAMP_P12] -> Sum11/2
  [TEST_P12] -> Sum11/1
  Sum11/1 -> P12_Out/1
  TEST_P13_In/1 -> [TEST_P13]
  TEST_P14_In/1 -> [TEST_P14]
  TEST_P15_In/1 -> [TEST_P15]
  TEST_P16_In/1 -> [TEST_P16]
  TEST_P17_In/1 -> [TEST_P17]
  TEST_P18_In/1 -> [TEST_P18]
  TEST_P19_In/1 -> [TEST_P19]
  TEST_P20_In/1 -> [TEST_P20]
  TEST_P21_In/1 -> [TEST_P21]
  TEST_P22_In/1 -> [TEST_P22]
  TEST_P23_In/1 -> [TEST_P23]
  TEST_P24_In/1 -> [TEST_P24]
  DAMP_P14_In/1 -> [DAMP_P14]
  DAMP_P13_In/1 -> [DAMP_P13]
  DAMP_P15_In/1 -> [DAMP_P15]
  DAMP_P17_In/1 -> [DAMP_P17]
  DAMP_P16_In/1 -> [DAMP_P16]
  DAMP_P18_In/1 -> [DAMP_P18]
  DAMP_P20_In/1 -> [DAMP_P20]
  DAMP_P19_In/1 -> [DAMP_P19]
  DAMP_P21_In/1 -> [DAMP_P21]
  DAMP_P23_In/1 -> [DAMP_P23]
  DAMP_P22_In/1 -> [DAMP_P22]
  DAMP_P24_In/1 -> [DAMP_P24]
  [DAMP_P13] -> Sum12/2
  [TEST_P13] -> Sum12/1
  Sum12/1 -> P13_Out/1
  [DAMP_P14] -> Sum13/2
  [TEST_P14] -> Sum13/1
  Sum13/1 -> P14_Out/1
  [DAMP_P15] -> Sum16/2
  [TEST_P15] -> Sum16/1
  Sum16/1 -> P15_Out/1
  [DAMP_P16] -> Sum17/2
  [TEST_P16] -> Sum17/1
  Sum17/1 -> P16_Out/1
  [DAMP_P17] -> Sum18/2
  [TEST_P17] -> Sum18/1
  Sum18/1 -> P17_Out/1
  [DAMP_P18] -> Sum19/2
  [TEST_P18] -> Sum19/1
  Sum19/1 -> P18_Out/1
  [DAMP_P19] -> Sum20/2
  [TEST_P19] -> Sum20/1
  Sum20/1 -> P19_Out/1
  [DAMP_P20] -> Sum21/2
  [TEST_P20] -> Sum21/1
  Sum21/1 -> P20_Out/1
  [DAMP_P21] -> Sum22/2
  [TEST_P21] -> Sum22/1
  Sum22/1 -> P21_Out/1
  [DAMP_P22] -> Sum23/2
  [TEST_P22] -> Sum23/1
  Sum23/1 -> P22_Out/1
  [DAMP_P23] -> Sum14/2
  [TEST_P23] -> Sum14/1
  Sum14/1 -> P23_Out/1
  [DAMP_P24] -> Sum24/2
  [TEST_P24] -> Sum24/1
  Sum24/1 -> P24_Out/1
